simulink model "Lab2_PW"  (R2018b)
settings: Solver=FixedStepAuto  StartTime=0.0  StopTime=1  FixedStep=0.001  RelTol=1e-3
libraries: cstblocks x6
settings Model: Creator=omeng  LastModifiedBy=omeng

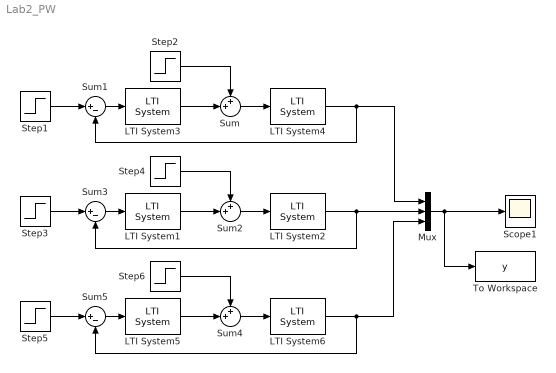
== system Lab2_PW ==
  LTI System1 : cstblocks/LTI System  sys=kc2  IC=[]
  LTI System2 : cstblocks/LTI System  sys=P  IC=[]
  LTI System3 : cstblocks/LTI System  sys=kc1  IC=[]
  LTI System4 : cstblocks/LTI System  sys=P  IC=[]
  LTI System5 : cstblocks/LTI System  sys=kc3  IC=[]
  LTI System6 : cstblocks/LTI System  sys=P  IC=[]
  Mux : Mux  Inputs=3
  Scope1 : Scope
  Step1 : Step  Time=0  SampleTime=0.001
  Step2 : Step  Time=0  After=0  SampleTime=0
  Step3 : Step  Time=0  SampleTime=0.001
  Step4 : Step  Time=0  After=0  SampleTime=0
  Step5 : Step  Time=0  SampleTime=0.001
  Step6 : Step  Time=0  After=0  SampleTime=0
  Sum : Sum  Inputs=++|
  Sum1 : Sum  Inputs=|+-
  Sum2 : Sum  Inputs=++|
  Sum3 : Sum  Inputs=|+-
  Sum4 : Sum  Inputs=++|
  Sum5 : Sum  Inputs=|+-
  To Workspace : ToWorkspace  VariableName=y  SaveFormat=Timeseries  SampleTime=-1
  wires:
  Step1/1 -> Sum1/1
  LTI System4/1 -> Sum1/2, Mux/1
  LTI System3/1 -> Sum/2
  Sum/1 -> LTI System4/1
  Step2/1 -> Sum/1
  Sum1/1 -> LTI System3/1
  Sum3/1 -> LTI System1/1
  Step4/1 -> Sum2/1
  Sum2/1 -> LTI System2/1
  LTI System1/1 -> Sum2/2
  LTI System2/1 -> Mux/2, Sum3/2
  Step3/1 -> Sum3/1
  Step5/1 -> Sum5/1
  LTI System6/1 -> Mux/3, Sum5/2
  LTI System5/1 -> Sum4/2
  Sum4/1 -> LTI System6/1
  Step6/1 -> Sum4/1
  Sum5/1 -> LTI System5/1
  Mux/1 -> Scope1/1, To Workspace/1
